simulink model "VE_Surveillance"  (R2021a)
settings: Solver=FixedStepAuto  StartTime=0.0  StopTime=2000  FixedStep=0.001  RelTol=1e-5
PreLoadFcn:
  | % ── Vecteurs de base ──────────────────────────────────────
  | SOC_vec = [0, 0.2, 0.4, 0.6, 0.8, 1.0];   % 6 points SOC
  | 
  | % Températures en KELVIN obligatoirement
  | T_vec = [273.15, 298.15, 318.15];          % 0°C, 25°C, 45°C
  | 
  | % ── V0(SOC,T) : matrice 6×3 ───────────────────────────────
  | % Lignes = SOC, Colonnes = T°
  | V0_table = [
  |     340, 345, 342;    % SOC = 0%
  |     355, 360, 357;    % SOC = 20%
  |     368, 373, 370;    % SOC = 40%
  |     380, 385, 382;    % SOC = 60%
  |     392, 397, 394;    % SOC = 80%
  |     400, 405, 402     % SOC = 100%
  | ];  % taille : 6×3 ✅
  | 
  | % ── R0(SOC,T) : matrice 6×3 ───────────────────────────────
  | R0_table = [
  |     0.08, 0.06, 0.07;   % SOC = 0%
  |     0.06, 0.05, 0.055;  % SOC = 20%
  |     0.05, 0.04, 0.045;  % SOC = 40%
  |     0.04, 0.03, 0.035;  % SOC = 60%
  |     0.04, 0.03, 0.035;  % SOC = 80%
  |     0.05, 0.04, 0.045   % SOC = 100%
  | ];  % taille : 6×3 ✅
  | 
  | % ── Capacité AH(T) : vecteur 1×3 ─────────────────────────
  | AH_vec = [55, 60, 62];   % Ah pour 0°C, 25°C, 45°C
libraries: fl_lib x8, nesl_utility x5, ee_lib x4, sdl_lib x1
(part 2 of 2)

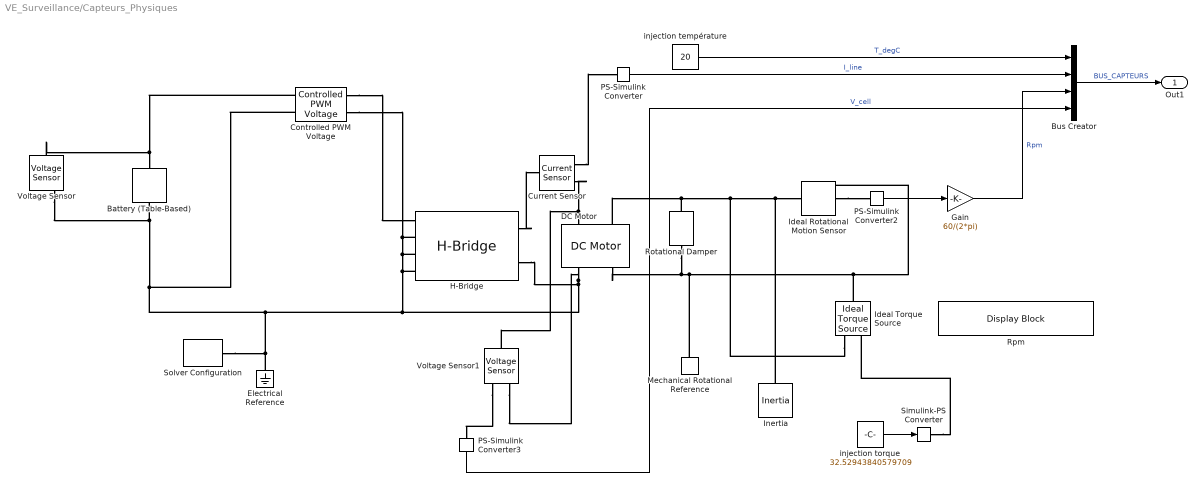
== system VE_Surveillance/Capteurs_Physiques ==
  Battery (Table-Based) : ee_lib/Sources/Battery (Table-Based)  SOC_vec=[0, 0.2, 0.4, 0.6, 0.8, 1.0]  T_dependence=ee.enum.temperature_dependence.yes  prm_dir=ee.enum.battery.prm_dir.noCurrentDirectionality  T_vec=[273.15, 298.15, 318.15] K  V0_mat=[340,345,342; 355,360,357; 368,373,370; 380,385,382; 392,397,394; 400,405,402] V  V0_vec=[3.1, 3.27, 3.31, 3.5] V  R0_mat=[0.08,0.06,0.07;0.06,0.05,0.055;0.05,0.04,0.045;0.04,0.03,0.035;0.04,0.03,0.035;0.05,0.04,0.045] Ohm  R0_vec=[.015, .017, .012, .013] Ohm  R0_dis_mat=[0.08, 0.06, 0.07; 0.06, 0.05, 0.055; 0.05, 0.04, 0.045; 0.04, 0.03, 0.035; 0.04, 0.03, 0.035; 0.05, 0.04, 0.045] Ohm  R0_dis_vec=[.015, .017, .012, .013] Ohm  R0_ch_mat=[0.08, 0.06, 0.07; 0.06, 0.05, 0.055; 0.05, 0.04, 0.045; 0.04, 0.03, 0.035; 0.04, 0.03, 0.035; 0.05, 0.04, 0.045] Ohm  R0_ch_vec=[.015, .017, .012, .013] Ohm  AH_vec=[55, 60, 62] hr*A  AH=4.1 hr*A  prm_leak=ee.enum.battery.prm_leak.enabled  Rleak_vec=[8000, 7000, 6000] Ohm  Rleak=7e3 Ohm  extrapolation_option=ee.enum.extrapolation.nearest  prm_dyn=ee.enum.battery.prm_dyn.off  R1_mat=[.089, .076, .01; .042, .022, .099; .019, .007, .002; .051, .043, .029] Ohm  R1_vec=[.076, .022, .007, .043] Ohm  tau1_mat=[44, 148, 235; 93, 110, 1000; 19, 27, 133; .5, 22, 3] s  tau1_vec=[148, 110, 27, 22] s  R2_mat=[.014, .382, .407; .028, .006, .007; .014, .007, .006; .333, .956, .912] Ohm  R2_vec=[.382, .006, .007, .956] Ohm  tau2_mat=[1, 44, 5644; 11, 24, 506; 2, 14, 330; 3310, 13419, 30216] s  tau2_vec=[44, 24, 14, 13419] s  R3_mat=[.014, .382, .407; .028, .006, .007; .014, .007, .006; .333, .956, .912] Ohm  R3_vec=[.382, .006, .007, .956] Ohm  tau3_mat=[1, 44, 5644; 11, 24, 506; 2, 14, 330; 3310, 13419, 30216] s  tau3_vec=[44, 24, 14, 13419] s  R4_mat=[.014, .382, .407; .028, .006, .007; .014, .007, .006; .333, .956, .912] Ohm  R4_vec=[.382, .006, .007, .956] Ohm  tau4_mat=[1, 44, 5644; 11, 24, 506; 2, 14, 330; 3310, 13419, 30216] s  tau4_vec=[44, 24, 14, 13419] s  R5_mat=[.014, .382, .407; .028, .006, .007; .014, .007, .006; .333, .956, .912] Ohm  R5_vec=[.382, .006, .007, .956] Ohm  tau5_mat=[1, 44, 5644; 11, 24, 506; 2, 14, 330; 3310, 13419, 30216] s  tau5_vec=[44, 24, 14, 13419] s  prm_fade=ee.enum.battery.prm_fade.equations  N0=100  dV0=0  dR0=0  dAH=0  dRleak=0  dR1=0  dR2=0  dR3=0  dR4=0  dR5=0  N0vec=[100, 200, 300]  Tfadevec=[298.15, 323.15] K  dV0vec=[0, 0, 0]  dR0vec=[0, 0, 0]  dAHvec=[0, 0, 0]  dRleakvec=[0, 0, 0]  dR1vec=[0, 0, 0]  dR2vec=[0, 0, 0]  dR3vec=[0, 0, 0]  dR4vec=[0, 0, 0]  dR5vec=[0, 0, 0]  dV0mat=[0, 0; 0, 0; 0, 0]  dR0mat=[0, 0; 0, 0; 0, 0]  dAHmat=[0, 0; 0, 0; 0, 0]  dRleakmat=[0, 0; 0, 0; 0, 0]  dR1mat=[0, 0; 0, 0; 0, 0]  dR2mat=[0, 0; 0, 0; 0, 0]  dR3mat=[0, 0; 0, 0; 0, 0]  dR4mat=[0, 0; 0, 0; 0, 0]  dR5mat=[0, 0; 0, 0; 0, 0]  prm_age=ee.enum.battery.prm_age.disabled  prm_age_OCV=ee.enum.battery.prm_age_OCV.OCV  OCV_age=0.9  SOC_age=0.6  storage_dt_age_vec=[0] d  storage_T_age_vec=[273] K  OCV_scaling_age=2.2134e6  OCV_offset_age=1.632e6  temp_exp_age=0.515833569 V  t_exp_age=0.75  T_age_vec=[273.15, 298.15, 323.15] K  dt_age_vec=[90, 180, 270, 360] d  dR0_age_vec=[0, 0, 0]  t_meas_dR0_age=100 d  dR0_age_mat=[0, 0, 0; 0, 0, 0; 0, 0, 0; 0, 0, 0]  temperature=298.15 K  i_specify=off  i_priority=None  i=0 A  i_nominal_specify=off  i_nominal_unit=A  i_nominal_value=1  v_specify=off  v_priority=None  v=0 V  v_nominal_specify=off  v_nominal_unit=V  v_nominal_value=1  stateOfCharge_specify=off  stateOfCharge_priority=High  stateOfCharge=1  stateOfCharge_nominal_specify=off  stateOfCharge_nominal_unit=1  stateOfCharge_nominal_value=1  num_cycles_specify=off  num_cycles_priority=High  num_cycles=0  num_cycles_nominal_specify=off  num_cycles_nominal_unit=1  num_cycles_nominal_value=1  thermal_mass=30000 J/K  temperature_specify=off  temperature_priority=High  temperature_nominal_specify=off  temperature_nominal_unit=K  temperature_nominal_value=1
      settings: SourceProductBaseCode=PS  InternalSimscapePortConfiguration="{\"Bottom\":[],\"Left\":[{\"id\":\"p\",\"label\":\"+\",\"type\":\"foundation.electrical.electrical\"}],\"Right\":[{\"id\":\"n\",\"label\":\"-\",\"type\":\"foundation.electrical.electrical\"}],\"Top\":[]}"
  Bus Creator : BusCreator  Inputs=4
  Controlled PWM Voltage : ee_lib/Integrated Circuits/Controlled PWM Voltage  F=1000 Hz  TD=0 s  pulse_width_offset=0 s  pulse_min=0 s  Vmin=0 V  Vmax=300 V  Vm=400 V  pwm_or_av=2  event_type=1  sample_time=1e-6 s  u_min=0  u_max=1
  Current Sensor : fl_lib/Electrical/Electrical Sensors/Current Sensor
  DC Motor : ee_lib/Electromechanical/Brushed Motors/DC Motor  field_option=ee.enum.field_option.pm  Rf=100 Ohm  Lf=1 H  Laf=0.15 H  If0=0 A  parameterization=ee.enum.dcparam_option.circuit_param  Ra=0.05 Ohm  La=12e-6 H  emf_or_torque=ee.enum.emf_or_torque.kv  Kv=0.05 V/rpm  Ki=6.876e-4 N*m/A  T_stall=0.24e-3 N*m  w_max=19100 rpm  w_rated=15000 rpm  P_rated=0.08 W  V_rated=1.5 V  J=0.05 kg*m^2  lam_param=ee.enum.lam_param.damping  lam=0 N*m/(rad/s)  i_noload=0 A  V_i_noload=1.5 V  speed0=0 rpm  enable_fault_armature=ee.enum.faults.faultEnable.no  rev_faulted=1 / 3  G_faulted_armature=1e-5 S  fault_trigger_armature=ee.enum.faults.faultTrigger.temporal  t_fault_armature=1 s  max_permissible_current_armature=inf A  t_fail_on_current_armature=1 s  enable_fault_field=ee.enum.faults.faultEnable.no  G_faulted_field=1e-5 S  fault_trigger_field=ee.enum.faults.faultTrigger.temporal  t_fault_field=1 s  max_permissible_current_field=inf A  t_fail_on_current_field=1 s  fault_action=ee.enum.faults.faultAction.none  alpha=3.93e-3 1/K  Tmeas=25 degC  thermal_mass=100 J/K  initial_temperature=25 degC
  Electrical Reference : fl_lib/Electrical/Electrical Elements/Electrical Reference
  Gain : Gain  Gain=60/(2*pi)
  H-Bridge : ee_lib/Semiconductors & Converters/Converters/H-Bridge  supply_ports=ee.enum.supply_ports.hidesupply  Venable=2.5 V  Vmax=5.0 V  Vreverse=2.5 V  Vbrake=2.5 V  Vm=12 V  pwm_or_av=ee.enum.pwm_or_av.averaged  regenerative_braking_mode=ee.enum.converters.regenerative_braking_mode.depends_on_rev  discontinuous=ee.enum.current_profile.continuous  freewheeling_mode=ee.enum.converters.freewheeling_mode.one_switch_one_diode  Ron=0.1 Ohm  Don=0.05 Ohm  Goff=1e-6 S  Rload=10 Ohm  Lload=1e-5 H  F=10 kHz  thermal_mass=100 J/K  initial_temperature=298.15 K  Ron2=0.1 Ohm  Don2=0.05 Ohm  Tmeas=298.15 K  Tmeas2=398.15 K
  Ideal Rotational Motion Sensor : fl_lib/Mechanical/Mechanical Sensors/Ideal Rotational Motion Sensor  wrap_angle=simscape.enum.onoff.off  offset=0 rad
  Ideal Torque Source : fl_lib/Mechanical/Mechanical Sources/Ideal Torque Source
  Inertia : fl_lib/Mechanical/Rotational Elements/Inertia  inertia=2 kg*m^2  num_ports=foundation.enum.numPorts2.one  w_specify=off  w_priority=High  w=0 rad/s  w_nominal_specify=off  w_nominal_unit=rad/s  w_nominal_value=1  t_specify=off  t_priority=None  t=0 N*m  t_nominal_specify=off  t_nominal_unit=N*m  t_nominal_value=1
  Mechanical Rotational Reference : fl_lib/Mechanical/Rotational Elements/Mechanical Rotational Reference
  PS-Simulink Converter : nesl_utility/PS-Simulink Converter  PhysicalDomain=network_engine_domain  SubClassName=ps_output  LeftPortType=input  RightPortType=output  PseudoPeriodic=off  Frequencies=[]  Unit=inherit  AffineConversion=off
      settings: SourceProductBaseCode=PW,SS
  PS-Simulink Converter2 : nesl_utility/PS-Simulink Converter  PhysicalDomain=network_engine_domain  SubClassName=ps_output  LeftPortType=input  RightPortType=output  PseudoPeriodic=off  Frequencies=[]  Unit=inherit  AffineConversion=off
      settings: SourceProductBaseCode=PW,SS
  PS-Simulink Converter3 : nesl_utility/PS-Simulink Converter  PhysicalDomain=network_engine_domain  SubClassName=ps_output  LeftPortType=input  RightPortType=output  PseudoPeriodic=off  Frequencies=[]  Unit=inherit  AffineConversion=off
      settings: SourceProductBaseCode=PW,SS
  Rotational Damper : sdl_lib/Couplings & Drives/Springs & Dampers/Rotational Damper  D=1e-3 N*m/(rad/s)  enable_faults=0  b_fault=100 N*m/(rad/s)  temporal_fault=0  fault_time=5 s  shock_fault=0  acceleration_limit=100 rad/s^2  shock_limit=1  report_fault=1
      settings: SourceProductBaseCode=LD
  Rpm : DisplayBlock  LabelPosition=Hide  Format=short  Transparency=1
  Simulink-PS Converter : nesl_utility/Simulink-PS Converter  PhysicalDomain=network_engine_domain  SubClassName=ps_input  LeftPortType=input  RightPortType=output  PseudoPeriodic=off  Frequencies=[]  NoiseDistribution=none  NoiseParameters=[]  Unit=N*m  AffineConversion=off  FilteringAndDerivatives=provide  SimscapeFilterOrder=1  InputFilterTimeConstant=0.001  UdotUserProvided=0
      settings: SourceProductBaseCode=PW,SS
  Solver Configuration : nesl_utility/Solver Configuration  PhysicalDomain=network_engine_domain  SubClassName=solver  LeftPortType=input  RightPortType=generic  Tones=[]  Harmonics=[]  SimulateNoise=off  Profile=off  UseLocalSampling=off  EnableSwitchedLinearOptims=on  FrequencyDomain=off  UseCCode=off  RelTol=0.001  AbsTol=1e-06  MinStep=1e-09  ToWorkspace=off  RevertToSquareIcSolve=off  NumHomotopyIterations=100  PhasorMode=off  PhasorModeNumHarmonics=1  DoDC=off  ResidualTolerance=1e-09  UseLocalSolver=on  LocalSolverChoice=NE_BACKWARD_EULER_ADVANCER  LocalSolverSampleTime=0.001  DoFixedCost=on  MaxNonlinIter=3  MaxModeIter=2  ComputeImpulses=off  ImpulseIterations=2  LinearAlgebra=auto  EquationFormulation=NE_TIME_EF  DelaysMemoryBudget=1024  AutomaticFiltering=on  FilteringTimeConstant=0.001  PartitionStorageMethod=AS_NEEDED  PartitionMemoryBudget=1024  PartitionMethod=ROBUST
      settings: SourceProductBaseCode=PW,SS
  Voltage Sensor : fl_lib/Electrical/Electrical Sensors/Voltage Sensor
  Voltage Sensor1 : fl_lib/Electrical/Electrical Sensors/Voltage Sensor
  injection température : Constant  Value=20
  injection torque : Constant  Value=32.52943840579709
  Out1 : Outport
  wires:
  PS-Simulink Converter/1 -> Bus Creator/2  "I_line"
  PS-Simulink Converter2/1 -> Gain/1
  injection température/1 -> Bus Creator/1  "T_degC"
  Gain/1 -> Bus Creator/3  "Rpm"
  Bus Creator/1 -> Out1/1  "BUS_CAPTEURS"
  injection torque/1 -> Simulink-PS Converter/1
  PS-Simulink Converter3/1 -> Bus Creator/4  "V_cell"
  connections:
  Voltage Sensor/LConn1 -- Controlled PWM Voltage/LConn1 -- Battery (Table-Based)/LConn1
  Voltage Sensor/RConn2 -- Voltage Sensor1/RConn2 -- DC Motor/RConn1 -- H-Bridge/RConn2 -- H-Bridge/LConn4 -- H-Bridge/LConn3 -- Controlled PWM Voltage/RConn2 -- H-Bridge/LConn2 -- Solver Configuration/RConn1 -- Electrical Reference/LConn1 -- Controlled PWM Voltage/LConn2 -- Battery (Table-Based)/RConn1
  Inertia/LConn1 -- DC Motor/LConn2 -- Rotational Damper/LConn1 -- Ideal Torque Source/RConn2 -- Ideal Rotational Motion Sensor/LConn1
  Ideal Rotational Motion Sensor/RConn2 -- PS-Simulink Converter2/LConn1
  Simulink-PS Converter/RConn1 -- Ideal Torque Source/RConn1
  Controlled PWM Voltage/RConn1 -- H-Bridge/LConn1
  H-Bridge/RConn1 -- Current Sensor/LConn1
  Current Sensor/RConn1 -- PS-Simulink Converter/LConn1
  Current Sensor/RConn2 -- Voltage Sensor1/LConn1 -- DC Motor/LConn1
  DC Motor/RConn2 -- Rotational Damper/RConn1 -- Mechanical Rotational Reference/LConn1 -- Ideal Torque Source/LConn1 -- Ideal Rotational Motion Sensor/RConn1
  Voltage Sensor1/RConn1 -- PS-Simulink Converter3/LConn1

== matlab function VE_Surveillance/Calcul_SOH ==
  data: N_cycles input; SOH output
function SOH = calcul_SOH(N_cycles)
    Q_initiale = 216000;
    taux = 0.0002;
    Q_actuelle = Q_initiale * (1 - taux * N_cycles);
    SOH = (Q_actuelle / Q_initiale) * 100;
    SOH = max(0, min(100, SOH));
end

== stateflow chart VE_Surveillance/BMS_VCU_Controller ==
  state Fault_Mode
    en: Vehicle_Mode = 4;
  state Normal_Mode
    en: Vehicle_Mode = 1;
  state Eco_Mode
    en: Vehicle_Mode = 2;
  state Alert_Mode
    en: Vehicle_Mode = 3;
  (default) -> Normal_Mode
  Alert_Mode -> Normal_Mode : [T_degC < 45 && SOC > 0.20]
  Normal_Mode -> Fault_Mode [order 3] : [T_degC >= 62 || SOC <= 0.05]
  Normal_Mode -> Alert_Mode [order 2] : [T_degC >= 50]
  Eco_Mode -> Normal_Mode [order 1] : [SOC > 0.25]
  Normal_Mode -> Eco_Mode [order 1] : [SOC <= 0.20]
  Eco_Mode -> Alert_Mode [order 2] : [T_degC >= 50]
  data: SOC input double; T_degC input double; Vehicle_Mode output uint8

== matlab function VE_Surveillance/MATLAB Function1 ==
  data: Puissance_kW input; Conso_inst output; Vitesse_kmh input
function Conso_inst = calc_conso_inst(Puissance_kW, Vitesse_kmh)
    % Sécurité : Si le véhicule est à l'arrêt ou roule à très faible vitesse
    if isnan(Puissance_kW) || isnan(Vitesse_kmh) || Vitesse_kmh < 0.5
        Conso_inst = 0; 
    else
        % Calcul de la consommation instantanée en kWh/100km
        Conso_inst = (Puissance_kW / Vitesse_kmh) * 100;
    end
end
